simulink model "LaboAPP3OldAsFuckForGaga"  (R2015b)
settings: Solver=VariableStepAuto  StartTime=0.0  StopTime=10.0  RelTol=1e-3
values from neighbouring files (symbols this model uses):
  A = [0 1 0 0; 0 0 0 0; 0 0 0 1; 0 0 0 0]    [App3.m]    (also in LaboratoireApp3.m; matlab.mat = [0 0 0 0 1 0 0 0 0 0 0 0 ... (16 elements, 4x4)])
  B = [0;-1;0;0]    [App3.m]    (also in LaboratoireApp3.m = [0;0;0;g]; matlab.mat = [0 -1 0 0])
  C = [1 0 0 0; 0 0 1 0]    [App3.m]    (also in LaboratoireApp3.m; matlab.mat = [1  0  0  0; 0  0  1  0])
  D = [0;0;]    [App3.m]    (also in LaboratoireApp3.m; matlab.mat = [0 0])
  frame = 1/24    (= 0.0416666666667)    [App3.m]    (also in LaboratoireApp3.m = 0.0333333333333; matlab.mat)
  init = [x,xdot,y,0]    [App3.m]    (also in LaboratoireApp3.m = [x;xdot;y;ydot]; matlab.mat = [14 1.5 2.50548611111 0])
  rayon = 1.5    [App3.m]    (also in matlab.mat)
  sol = 1    [App3.m]    (also in LaboratoireApp3.m = 10; matlab.mat)
settings Model: Creator=spip2401  LastModifiedBy=Philippe
settings DataIOCC: LimitDataPoints=off
settings DebuggingCC: AllowSymbolicDim=on
settings ModelReferenceCC: PropagateSignalLabelsOutOfModel=on
settings GRTTargetCC: GeneratePreprocessorConditionals=Disable all
settings ConfigComp: CovModelRefEnable=Off

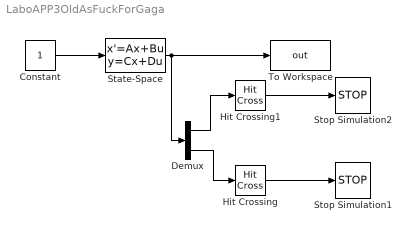
== system LaboAPP3OldAsFuckForGaga ==
  Constant : Constant
  Demux : Demux  Outputs=2
  Hit Crossing : HitCross  HitCrossingOffset=sol + rayon  HitCrossingDirection=falling
  Hit Crossing1 : HitCross  HitCrossingOffset=15
  State-Space : StateSpace  A=A  B=B  C=C  D=D  X0=init
  Stop Simulation1 : Stop
  Stop Simulation2 : Stop
  To Workspace : ToWorkspace  VariableName=out  SaveFormat=Timeseries  SampleTime=frame
  wires:
  Constant/1 -> State-Space/1
  State-Space/1 -> Demux/1, To Workspace/1
  Demux/2 -> Hit Crossing/1
  Hit Crossing/1 -> Stop Simulation1/1
  Hit Crossing1/1 -> Stop Simulation2/1
  Demux/1 -> Hit Crossing1/1
